simulink model "simulacaoisaqueMIC2"  (R2023a)
settings: Solver=VariableStepAuto  StartTime=0.0  StopTime=2  RelTol=1e-3
libraries: instrumentlib x8, cstblocks x4
settings Model: Creator=Aluno - LPR 6  LastModifiedBy=Aluno - LPR 6

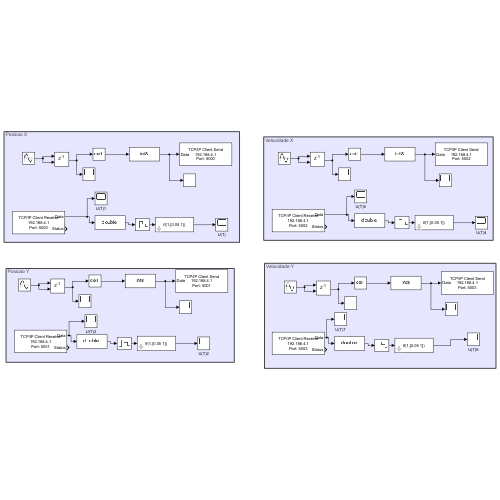
[thumbnail: Simulink's stored preview of the top-level diagram]
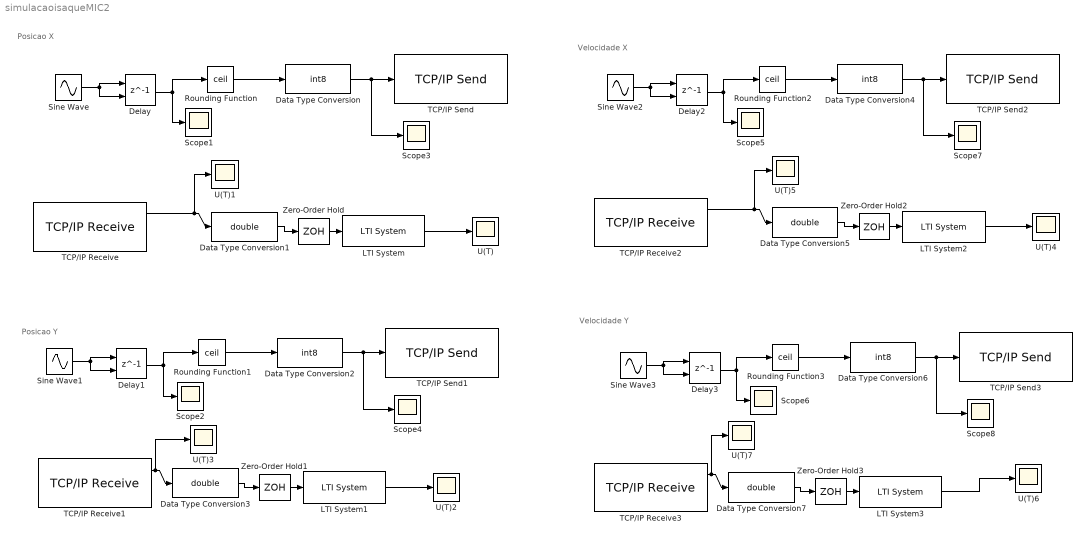
== system simulacaoisaqueMIC2 ==
  note: Velocidade Y
  note: Velocidade X
  note: Posicao Y
  note: Posicao X
  Data Type Conversion{,2,4,6} (4 alike) : DataTypeConversion  OutDataTypeStr=int8  SaturateOnIntegerOverflow=off  RndMeth=Floor
  Data Type Conversion{1,3,5,7} (4 alike) : DataTypeConversion  OutDataTypeStr=double  SaturateOnIntegerOverflow=off  RndMeth=Floor
  Delay{,1..3} (4 alike) : Delay  DelayLength=1  InitialConditionSource=Input port  InitialCondition=0
      settings: InputPortMap=u0,p4
  LTI System{,1..3} (4 alike) : cstblocks/LTI System  sys=tf(1,[0.05 1])  IC=[]
  Rounding Function{,1..3} (4 alike) : Rounding  Operator=ceil
  Scope{1..8} (8 alike) : Scope
  Sine Wave : Sin  Amplitude=150  Frequency=2  SampleTime=0
  Sine Wave1 : Sin  Amplitude=150  Frequency=2  Phase=2  SampleTime=0
  Sine Wave2 : Sin  Amplitude=150  Frequency=2  SampleTime=0
  Sine Wave3 : Sin  Amplitude=150  Frequency=2  Phase=2  SampleTime=0
  TCP/IP Receive : instrumentlib/TCP//IP Receive  Host=192.168.4.1  Port=5000  DataSize=[ 1, 1 ]  DataType=int8  ASCIIFormatting=%f  Terminator=CR  CustomTerminator=10  ByteOrder=big-endian  EnableBlockingMode=off  Timeout=10  SampleTime=0.0001  SimulateUsing=Interpreted execution
  TCP/IP Receive1 : instrumentlib/TCP//IP Receive  Host=192.168.4.1  Port=5001  DataSize=[ 1, 1 ]  DataType=int8  ASCIIFormatting=%f  Terminator=CR  CustomTerminator=10  ByteOrder=big-endian  EnableBlockingMode=off  Timeout=10  SampleTime=0.0001  SimulateUsing=Interpreted execution
  TCP/IP Receive2 : instrumentlib/TCP//IP Receive  Host=192.168.4.1  Port=5002  DataSize=[ 1, 1 ]  DataType=int8  ASCIIFormatting=%f  Terminator=CR  CustomTerminator=10  ByteOrder=big-endian  EnableBlockingMode=off  Timeout=10  SampleTime=0.0001  SimulateUsing=Interpreted execution
  TCP/IP Receive3 : instrumentlib/TCP//IP Receive  Host=192.168.4.1  Port=5003  DataSize=[ 1, 1 ]  DataType=int8  ASCIIFormatting=%f  Terminator=CR  CustomTerminator=10  ByteOrder=big-endian  EnableBlockingMode=off  Timeout=10  SampleTime=0.0001  SimulateUsing=Interpreted execution
  TCP/IP Send : instrumentlib/TCP//IP Send  Host=192.168.4.1  Port=5000  ByteOrder=big-endian  EnableBlockingMode=off  Timeout=10  TransferDelay=on  SimulateUsing=Interpreted execution
  TCP/IP Send1 : instrumentlib/TCP//IP Send  Host=192.168.4.1  Port=5001  ByteOrder=big-endian  EnableBlockingMode=off  Timeout=10  TransferDelay=on  SimulateUsing=Interpreted execution
  TCP/IP Send2 : instrumentlib/TCP//IP Send  Host=192.168.4.1  Port=5002  ByteOrder=big-endian  EnableBlockingMode=off  Timeout=10  TransferDelay=on  SimulateUsing=Interpreted execution
  TCP/IP Send3 : instrumentlib/TCP//IP Send  Host=192.168.4.1  Port=5003  ByteOrder=big-endian  EnableBlockingMode=off  Timeout=10  TransferDelay=on  SimulateUsing=Interpreted execution
  U(T){,1..7} (8 alike) : Scope
  Zero-Order Hold{,1..3} (4 alike) : ZeroOrderHold  SampleTime=0.0001
  wires:
  TCP/IP Receive/1 -> U(T)1/1, Data Type Conversion1/1
  Data Type Conversion1/1 -> Zero-Order Hold/1
  Data Type Conversion/1 -> Scope3/1, TCP/IP Send/1
  Rounding Function/1 -> Data Type Conversion/1
  LTI System/1 -> U(T)/1
  Delay/1 -> Rounding Function/1, Scope1/1
  Zero-Order Hold/1 -> LTI System/1
  Sine Wave/1 -> Delay/1, Delay/2
  Delay1/1 -> Rounding Function1/1, Scope2/1
  Rounding Function1/1 -> Data Type Conversion2/1
  LTI System1/1 -> U(T)2/1
  Data Type Conversion3/1 -> Zero-Order Hold1/1
  Zero-Order Hold1/1 -> LTI System1/1
  TCP/IP Receive1/1 -> U(T)3/1, Data Type Conversion3/1
  Sine Wave1/1 -> Delay1/1, Delay1/2
  Data Type Conversion2/1 -> Scope4/1, TCP/IP Send1/1
  LTI System3/1 -> U(T)6/1
  LTI System2/1 -> U(T)4/1
  Data Type Conversion7/1 -> Zero-Order Hold3/1
  Sine Wave3/1 -> Delay3/1, Delay3/2
  Data Type Conversion6/1 -> Scope8/1, TCP/IP Send3/1
  Data Type Conversion4/1 -> Scope7/1, TCP/IP Send2/1
  Rounding Function3/1 -> Data Type Conversion6/1
  Rounding Function2/1 -> Data Type Conversion4/1
  Sine Wave2/1 -> Delay2/1, Delay2/2
  TCP/IP Receive2/1 -> U(T)5/1, Data Type Conversion5/1
  Data Type Conversion5/1 -> Zero-Order Hold2/1
  Delay3/1 -> Rounding Function3/1, Scope6/1
  Delay2/1 -> Rounding Function2/1, Scope5/1
  TCP/IP Receive3/1 -> U(T)7/1, Data Type Conversion7/1
  Zero-Order Hold3/1 -> LTI System3/1
  Zero-Order Hold2/1 -> LTI System2/1
